simulink model "E010A5_C0_baseline_40A_1A_20260630"  (R2024b)
settings: Solver=VariableStepAuto  StartTime=0.0  StopTime=0.54e-3  MaxStep=5e-9  RelTol=1e-3
undefined symbols (not defined in the file): A_init, A_lower, A_upper, Cout, DCR_L1, DCR_L2, DCR_L3, DCR_L4, E010A5_DeltaI_Drop_Threshold_High, E010A5_IL_Sense_Gain1, E010A5_IL_Sense_Gain2, E010A5_IL_Sense_Gain3, E010A5_IL_Sense_Gain4, ESR_C, IdealIQCOT_Enable, IL_adc_counts_per_A, IL_pk_limit_adc_neg, IL_pk_limit_adc_pos, Iload_final, Iload_initial, Iph, Iqcot_enable, kappa_cmd, Kiqcot, Kvc_iqcot, L, Lambda0_iqcot, Lambda_m2, rho_cmd, Ri_iqcot, t_load_step, Tblank, Tdead, Tiqcot_leak, Toff_min, Ton_cmd, Ton_iq_max, Ton_iq_min, Ts_ctrl, Tslot, Tss, Vc_bias_iqcot, Vcot_ramp_amp, Vcot_ramp_enable, Vhys, Vin, Vo_ref
libraries: simulink x29, spsCurrentMeasurementLib x8, spsMosfetLib x8, spsSeriesRLCBranchLib x5, spsVoltageMeasurementLib x5, spsDCVoltageSourceLib x4, spsControlledCurrentSourceLib x1, spsGroundLib x1, spspowerguiLib x1
(part 1 of 2)
settings Model: Creator=zengruize  LastModifiedBy=zengruize

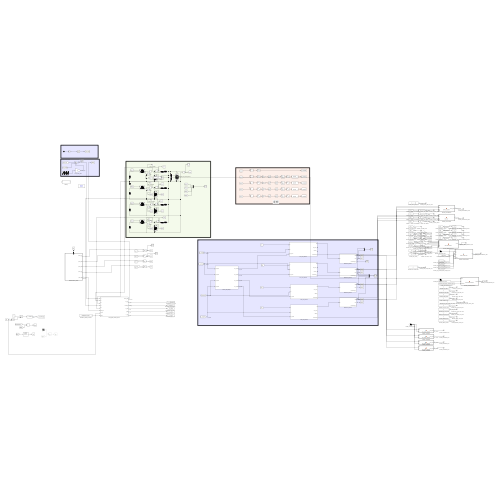
[thumbnail: Simulink's stored preview of the top-level diagram]
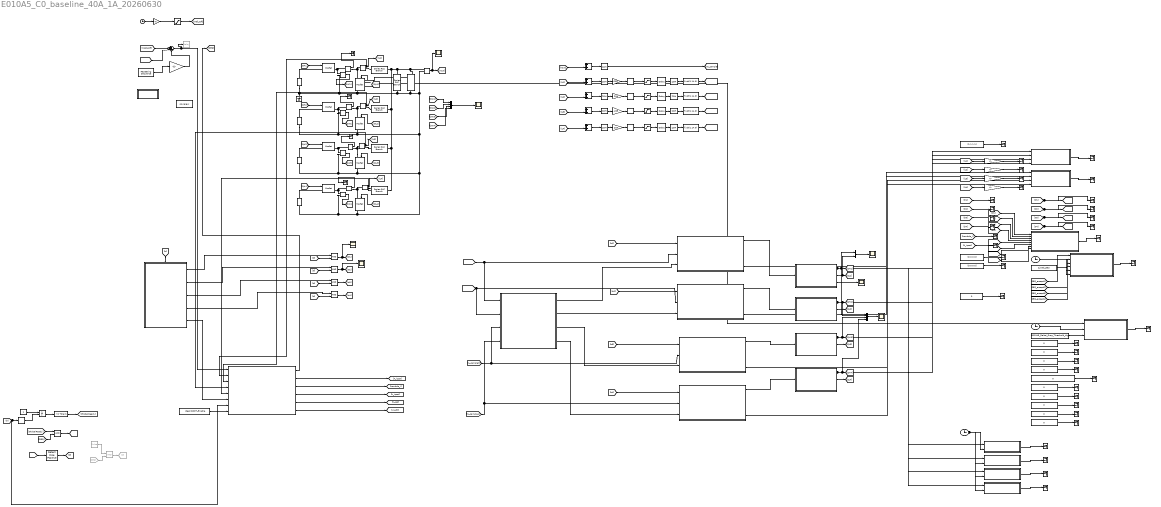
== system E010A5_C0_baseline_40A_1A_20260630 ==
  note: cot
  note: 输出电压误差比较器
  note: 功率级
  note: 软启动
  note: 采样
  Add{,1..4} (5 alike) : Sum
  Bus Creator : BusCreator  Inputs=4
  Bus Creator1 : BusCreator  Inputs=2
  Bus Creator2 : BusCreator  Inputs=4
  COT_Cell_1Phase1 : Subsystem
  COT_Cell_1Phase2 : Subsystem
  COT_Cell_1Phase3 : Subsystem
  COT_Cell_1Phase4 : Subsystem
  Clock : Clock
  Compare To Constant : simulink/Logic and Bit Operations/Compare To Constant  relop=>=  const=Tblank  OutDataTypeStr=boolean
  Constant : Constant
  Current Measurement{,1..3} (4 alike) : spsCurrentMeasurementLib/Current Measurement  PhasorSimulation=off  OutputType=Complex  PSBequivalent=0
  DC Voltage Source{,1..3} (4 alike) : spsDCVoltageSourceLib/DC Voltage Source  Amplitude=Vin  Measurements=None
  Data Type Conversion{,2..4} (4 alike) : DataTypeConversion  OutDataTypeStr=fixdt(1,14,0)  SaturateOnIntegerOverflow=off  RndMeth=Floor
  Detect Rise Positive : simulink/Logic and Bit Operations/Detect Rise Positive  vinit=0  OutDataTypeStr=boolean
  E010A5_ActiveHSPhase : MATLAB Function  TreatAsAtomicUnit=on
  E010A5_ActiveHSPhase_Term : Terminator
  E010A5_CurrentLimitHit : MATLAB Function  TreatAsAtomicUnit=on
  E010A5_CurrentLimitHit_Term : Terminator
  E010A5_IL_Sense_Gain_Block1 : Gain  Gain=E010A5_IL_Sense_Gain1
  E010A5_IL_Sense_Gain_Block2 : Gain  Gain=E010A5_IL_Sense_Gain2
  E010A5_IL_Sense_Gain_Block3 : Gain  Gain=E010A5_IL_Sense_Gain3
  E010A5_IL_Sense_Gain_Block4 : Gain  Gain=E010A5_IL_Sense_Gain4
  E010A5_IL_Sense_Term{1..4} (4 alike) : Terminator
  E010A5_LoadCurrentStep : Step  Time=t_load_step  Before=Iload_initial  After=Iload_final  SampleTime=0
  E010A5_Load_Current_Source : spsControlledCurrentSourceLib/Controlled Current Source  Initialize=on  Source_Type=DC  Amplitude=0  Phase=0  Frequency=0  Measurements=None
  E010A5_Log_Lambda_i_Term : Terminator
  E010A5_Log_REQ1_Term : Terminator
  E010A5_Log_REQ2_Term : Terminator
  E010A5_Log_REQ3_Term : Terminator
  E010A5_Log_REQ4_Term : Terminator
  E010A5_Log_area_int_i_Term : Terminator
  E010A5_PhaseOrderError : MATLAB Function  TreatAsAtomicUnit=on  SystemSampleTime=Ts_ctrl
  E010A5_PhaseOrderError_Term : Terminator
  E010A5_PhaseOrder_Clock : Clock
  E010A5_PhaseOrder_LoadStepTime : Constant  Value=t_load_step
  E010A5_REQAccept_Term{1..4} (4 alike) : Terminator
  E010A5_REQRejectReason : MATLAB Function  TreatAsAtomicUnit=on
  E010A5_REQRejectReason_Term : Terminator
  E010A5_SevereDropDetector : MATLAB Function  TreatAsAtomicUnit=on  SystemSampleTime=Ts_ctrl
  E010A5_SevereDropDetector_Clock : Clock
  E010A5_SevereDropDetector_Term : Terminator
  E010A5_SevereDropThreshold : Constant  Value=E010A5_DeltaI_Drop_Threshold_High
  E010A5_TonActual1 : MATLAB Function  TreatAsAtomicUnit=on  SystemSampleTime=Ts_ctrl
  E010A5_TonActual1_Term : Terminator
  E010A5_TonActual2 : MATLAB Function  TreatAsAtomicUnit=on  SystemSampleTime=Ts_ctrl
  E010A5_TonActual2_Term : Terminator
  E010A5_TonActual3 : MATLAB Function  TreatAsAtomicUnit=on  SystemSampleTime=Ts_ctrl
  E010A5_TonActual3_Term : Terminator
  E010A5_TonActual4 : MATLAB Function  TreatAsAtomicUnit=on  SystemSampleTime=Ts_ctrl
  E010A5_TonActual4_Term : Terminator
  E010A5_TonActual_Clock : Clock
  E010A5_Ton_saved_i : Constant  Value=[0 0 0 0]
  E010A5_Ton_saved_i_Term : Terminator
  E010A5_Ton_trunc_i : Constant  Value=[0 0 0 0]
  E010A5_Ton_trunc_i_Term : Terminator
  E010A5_a_O_state : Constant  Value=0
  E010A5_a_O_state_Term : Terminator
  E010A5_active_phase_set : Constant  Value=[1 1 1 1]
  E010A5_active_phase_set_Term : Terminator
  E010A5_area_bleed_count : Constant  Value=0
  E010A5_area_bleed_count_Term : Terminator
  E010A5_area_hold_count : Constant  Value=0
  E010A5_area_hold_count_Term : Terminator
  E010A5_area_hold_state : Constant  Value=0
  E010A5_area_hold_state_Term : Terminator
  E010A5_area_reset_count : Constant  Value=0
  E010A5_area_reset_count_Term : Terminator
  E010A5_burst_pulse_count_after_reentry : Constant  Value=0
  E010A5_burst_pulse_count_after_reentry_Term : Terminator
  E010A5_fallback_count : Constant  Value=0
  E010A5_fallback_count_Term : Terminator
  E010A5_fallback_reason : Constant  Value=0
  E010A5_fallback_reason_Term : Terminator
  E010A5_fallback_state : Constant  Value=0
  E010A5_fallback_state_Term : Terminator
  E010A5_pulse_inhibit_state : Constant  Value=0
  E010A5_pulse_inhibit_state_Term : Terminator
  E010A5_reentry_state : Constant  Value=0
  E010A5_reentry_state_Term : Terminator
  From31 : From  Commented=on  GotoTag=REQ
  Gain : Gain  Gain=Vo_ref / Tss
  Gain11 : Gain  Gain=205
  Gain12 : Gain  Gain=-205
  Gain13 : Gain  Gain=205
  Gain9 : Gain  Gain=-205
  GateDriver_1Phase1 : Subsystem
  GateDriver_1Phase2 : Subsystem
  GateDriver_1Phase3 : Subsystem
  GateDriver_1Phase4 : Subsystem
  Goto26 : Goto  Commented=on  GotoTag=tr
  Ground : spsGroundLib/Ground  LConnTagsString=a
  IHS_Terminator{1..4} (4 alike) : Terminator
  IL_Measurement{1..4} (4 alike) : spsCurrentMeasurementLib/Current Measurement  PhasorSimulation=off  OutputType=Complex  PSBequivalent=0
  IQCOT_Ton_Adapter : Subsystem
  IdealIQCOT_Enable_Constant : Constant  Value=IdealIQCOT_Enable
  Ideal_Digital_IQCOT_Request : Subsystem
  Integrator : Integrator  ExternalReset=rising
  Logical Operator{,1..4} (5 alike) : Logic  AllPortsSameDT=off  OutDataTypeStr=boolean
  Logical Operator5 : Logic  Commented=on  AllPortsSameDT=off  OutDataTypeStr=boolean
  Memory : Memory
  Mosfet{,1..3} (4 alike) : spsMosfetLib/Mosfet  Ron=Ron_HS  Lon=0  Rd=Rd_body  Vfd=Vfd_body  IC=0  Rs=Rs_snubber  Cs=Cs_snubber  Measurements=on
  Mosfet{4..7} (4 alike) : spsMosfetLib/Mosfet  Ron=Ron_LS  Lon=0  Rd=Rd_body  Vfd=Vfd_body  IC=0  Rs=Rs_snubber  Cs=Cs_snubber  Measurements=on
  OnDelay : Subsystem
  PhaseScheduler_4Phase : Subsystem  TreatAsAtomicUnit=on
  Pulse Generator : DiscretePulseGenerator  Commented=on  PulseType=Time based  Period=Tblank  PulseWidth=5
  Quantizer{1..4} (4 alike) : Quantizer  QuantizationInterval=1
  Relay : Relay  Commented=through  OnSwitchValue=Vhys/2  OffSwitchValue=-Vhys/2
  Saturation{,1,3..4} (4 alike) : Saturate  UpperLimit=8191  LowerLimit=-8191
  Saturation2 : Saturate  UpperLimit=Vo_ref  LowerLimit=0
  Scope{,1..6} (7 alike) : Scope
  Series RLC Branch : spsSeriesRLCBranchLib/Series RLC Branch  LConnTagsString=__new0  RConnTagsString=__new0  BranchType=RL  Resistance=DCR_L1  Inductance=L  SetiL0=off  InitialCurrent=0  Capacitance=1e-6  Setx0=off  InitialVoltage=0  Measurements=None
  Series RLC Branch1 : spsSeriesRLCBranchLib/Series RLC Branch  LConnTagsString=__new0  RConnTagsString=__new0  BranchType=RL  Resistance=DCR_L2  Inductance=L  SetiL0=off  InitialCurrent=0  Capacitance=1e-6  Setx0=off  InitialVoltage=0  Measurements=None
  Series RLC Branch2 : spsSeriesRLCBranchLib/Series RLC Branch  LConnTagsString=__new0  RConnTagsString=__new0  BranchType=RL  Resistance=DCR_L3  Inductance=L  SetiL0=off  InitialCurrent=0  Capacitance=1e-6  Setx0=off  InitialVoltage=0  Measurements=None
  Series RLC Branch3 : spsSeriesRLCBranchLib/Series RLC Branch  LConnTagsString=__new0  RConnTagsString=__new0  BranchType=RL  Resistance=DCR_L4  Inductance=L  SetiL0=off  InitialCurrent=0  Capacitance=1e-6  Setx0=off  InitialVoltage=0  Measurements=None
  Series RLC Branch4 : spsSeriesRLCBranchLib/Series RLC Branch  LConnTagsString=__new0  RConnTagsString=__new0  BranchType=RC  Resistance=ESR_C  Inductance=1e-3  SetiL0=off  InitialCurrent=0  Capacitance=Cout  Setx0=on  InitialVoltage=Vo_ref  Measurements=None
  Sum : Sum  Inputs=|+--
  Transport Delay{1..4} (4 alike) : TransportDelay  DelayTime=5/25000000
  VCOT_Ramp_Gain : Gain  Gain=Vcot_ramp_enable * Vcot_ramp_amp
  VCOT_Ramp_Unit : simulink/Sources/Repeating Sequence  rep_seq_t=[0 Tslot]  rep_seq_y=[0 1]
  Voltage Measurement{,1..4} (5 alike) : spsVoltageMeasurementLib/Voltage Measurement  PhasorSimulation=off  OutputType=Complex  PSBequivalent=0
  Zero-Order Hold{1..4,19..23} (9 alike) : ZeroOrderHold  SampleTime=1/25000000
  powergui : spspowerguiLib/powergui  Priority=1  SimulationMode=Discrete  SampleTime=2e-9  frequency=60  Iterations=50  frequencyindice=0  Pbase=100e6  ErrMax=1e-4  UnitsV=kV  UnitsW=MW  buscounter=0  FunctionMessages=off  echomessages=off  EnableUseOfTLC=off  CurrentSourceSwitches=off  DisableSnubberDevices=off  DisableRonSwitches=off  DisableVfSwitches=off  DisplayEquations=off  AutomaticDiscreteSolvers=off  SolverType=Tustin/Backward Euler (TBE)  Interpol=off  ExternalGateDelay=off  methode=off  Ts=100  x0status=blocks  SPID=on  SwTol=0  HookPort=off  NonlinearTolerance=1e-4  nMaxIteration=100  ContinueOnMaxIteration=off  RestoreLinks=warning  ResistiveCurrentMeasurement=off  Frange=[0:2:500]  Ylog=off  Xlog=on  ShowGrid=off  save=off  variable=ZData  structure=0  ZoomFFT=off  StartTime=0.0  cycles=1  DisplayStyle=1  fundamental=60  FreqAxis=off  MaxFrequency=1000  frequencyindicesteady=1  RmsSteady=1  display=off
  wires:
  [QH1] -> Mosfet/1
  [QH4] -> Mosfet3/1
  [QH2] -> Mosfet1/1
  [QH3] -> Mosfet2/1
  [QL1] -> Mosfet4/1
  [QL2] -> Mosfet5/1
  [QL3] -> Mosfet6/1
  [QL4] -> Mosfet7/1
  Voltage Measurement2/1 -> [SW2]  "SW2"
  Voltage Measurement3/1 -> [SW3]  "SW3"
  Voltage Measurement1/1 -> [SW1]  "SW1"
  Voltage Measurement4/1 -> [SW4]  "SW4"
  GateDriver_1Phase1/1(QHi) -> Bus Creator1/1, [QH1], Bus Creator2/1, E010A5_ActiveHSPhase/1(qh1), E010A5_TonActual1/1(qh)  "QH1"
  GateDriver_1Phase2/1(QHi) -> Bus Creator2/2, [QH2], E010A5_ActiveHSPhase/2(qh2), E010A5_TonActual2/1(qh)  "QH2"
  GateDriver_1Phase3/1(QHi) -> Bus Creator2/3, [QH3], E010A5_ActiveHSPhase/3(qh3), E010A5_TonActual3/1(qh)  "QH3"
  GateDriver_1Phase4/1(QHi) -> Bus Creator2/4, [QH4], E010A5_ActiveHSPhase/4(qh4), E010A5_TonActual4/1(qh)  "QH4"
  GateDriver_1Phase1/2(QLi) -> Bus Creator1/2, [QL1]  "QL1"
  GateDriver_1Phase2/2(QLi) -> [QL2]  "QL2"
  GateDriver_1Phase3/2(QLi) -> [QL3]  "QL3"
  GateDriver_1Phase4/2(QLi) -> [QL4]  "QL4"
  COT_Cell_1Phase1/1(Qi) -> GateDriver_1Phase1/1(Qi)
  COT_Cell_1Phase2/1(Qi) -> GateDriver_1Phase2/1(Qi)
  COT_Cell_1Phase3/1(Qi) -> GateDriver_1Phase3/1(Qi)
  COT_Cell_1Phase4/1(Qi) -> GateDriver_1Phase4/1(Qi)
  GateDriver_1Phase1/3(ShootThrough_i) -> Scope1/1
  Bus Creator/1 -> Scope2/1
  [SW1] -> Bus Creator/1
  [SW2] -> Bus Creator/2
  [SW3] -> Bus Creator/3
  [SW4] -> Bus Creator/4
  Bus Creator1/1 -> Scope3/1
  Saturation2/1 -> [Vref_soft]
  Gain/1 -> Saturation2/1
  Clock/1 -> Gain/1
  Voltage Measurement/1 -> Scope/1, [Vout]  "Vout"
  [Vref_soft] -> Sum/1
  [Vo_sample] -> Sum/2
  Sum/1 -> Ideal_Digital_IQCOT_Request/1(e_v), Relay/1  "e_v"
  Constant/1 -> Integrator/1
  Integrator/1 -> Compare To Constant/1
  Compare To Constant/1 -> [GlobalReady]  "Allow"
  [GlobalReady] -> Logical Operator/1
  [REQ] -> Logical Operator/2
  Logical Operator/1 -> [Allow]
  [Allow] -> Detect Rise Positive/1
  Detect Rise Positive/1 -> [tr]
  [tr] -> PhaseScheduler_4Phase/Trigger  "tr"
  PhaseScheduler_4Phase/1(phase_en1) -> Logical Operator1/1
  [tr] -> Logical Operator1/2
  PhaseScheduler_4Phase/2(phase_en2) -> Logical Operator2/1
  [tr] -> Logical Operator2/2
  PhaseScheduler_4Phase/3(phase_en3) -> Logical Operator3/1
  [tr] -> Logical Operator3/2
  PhaseScheduler_4Phase/4(phase_en4) -> Logical Operator4/1
  [tr] -> Logical Operator4/2
  Logical Operator1/1 -> Scope4/1, [tr1]  "tr1"
  Logical Operator2/1 -> Scope5/1, [tr2]  "tr2"
  Logical Operator3/1 -> [tr3]  "tr3"
  Logical Operator4/1 -> [tr4]  "tr4"
  [tr1] -> COT_Cell_1Phase1/1(tri)
  [tr2] -> COT_Cell_1Phase2/1(tri)
  [tr3] -> COT_Cell_1Phase3/1(tri)
  [tr4] -> COT_Cell_1Phase4/1(tri)
  [IL_sample1] -> COT_Cell_1Phase1/2(ILi), IQCOT_Ton_Adapter/1(IL_sample1)  "IL_sample1"
  [IL_sample2] -> IQCOT_Ton_Adapter/2(IL_sample2), COT_Cell_1Phase2/2(ILi)  "IL_sample2"
  [IL_sample3] -> IQCOT_Ton_Adapter/3(IL_sample3), COT_Cell_1Phase3/2(ILi)  "IL_sample3"
  [IL_sample4] -> IQCOT_Ton_Adapter/4(IL_sample4), COT_Cell_1Phase4/2(ILi)  "IL_sample4"
  [tr] -> Memory/1, Ideal_Digital_IQCOT_Request/7(tr_reset)  "tr_reset"
  Memory/1 -> Integrator/2
  Logical Operator5/1 -> Goto26/1
  Pulse Generator/1 -> Logical Operator5/1
  From31/1 -> Logical Operator5/2
  Bus Creator2/1 -> Scope6/1
  IL_Measurement1/1 -> [IL1], Ideal_Digital_IQCOT_Request/2(IL1)  "IL1"
  IL_Measurement2/1 -> [IL2], Ideal_Digital_IQCOT_Request/3(IL2)  "IL2"
  IL_Measurement3/1 -> [IL3], Ideal_Digital_IQCOT_Request/4(IL3)  "IL3"
  IL_Measurement4/1 -> [IL4], Ideal_Digital_IQCOT_Request/5(IL4)  "IL4"
  Current Measurement/1 -> IHS_Terminator1/1
  Current Measurement1/1 -> IHS_Terminator2/1
  Current Measurement2/1 -> IHS_Terminator3/1
  Current Measurement3/1 -> IHS_Terminator4/1
  Zero-Order Hold23/1 -> Gain13/1
  Zero-Order Hold20/1 -> Gain9/1
  Zero-Order Hold3/1 -> Data Type Conversion3/1
  Zero-Order Hold4/1 -> Data Type Conversion2/1
  Saturation4/1 -> Transport Delay4/1
  Zero-Order Hold1/1 -> Data Type Conversion/1
  [IL3] -> Add3/2
  Add3/1 -> Zero-Order Hold22/1
  Quantizer1/1 -> Saturation/1
  Quantizer4/1 -> Saturation4/1
  Gain12/1 -> Quantizer3/1
  [IL4] -> Add4/2
  Add/1 -> Zero-Order Hold19/1
  Data Type Conversion/1 -> [IL_sample1]
  Data Type Conversion2/1 -> [IL_sample4]
  Add4/1 -> Zero-Order Hold23/1
  Transport Delay3/1 -> Zero-Order Hold3/1
  Saturation3/1 -> Transport Delay3/1
  Add1/1 -> Zero-Order Hold20/1
  [IL1] -> Add1/2
  Transport Delay4/1 -> Zero-Order Hold4/1
  Zero-Order Hold21/1 -> Gain11/1
  Data Type Conversion3/1 -> [IL_sample3]
  Gain9/1 -> Quantizer1/1
  Gain11/1 -> Quantizer2/1
  Saturation/1 -> Transport Delay1/1
  [IL2] -> Add2/2
  Transport Delay2/1 -> Zero-Order Hold2/1
  Zero-Order Hold19/1 -> [Vo_sample]
  Gain13/1 -> Quantizer4/1
  Quantizer3/1 -> Saturation3/1
  Data Type Conversion4/1 -> [IL_sample2]
  Zero-Order Hold2/1 -> Data Type Conversion4/1
  Add2/1 -> Zero-Order Hold21/1
  Transport Delay1/1 -> Zero-Order Hold1/1
  [Vout] -> Add/2
  Saturation1/1 -> Transport Delay2/1
  Zero-Order Hold22/1 -> Gain12/1
  Quantizer2/1 -> Saturation1/1
  VCOT_Ramp_Unit/1 -> VCOT_Ramp_Gain/1
  VCOT_Ramp_Gain/1 -> Sum/3  "Vcot_ramp"
  IQCOT_Ton_Adapter/1(Ton_iqcot1) -> COT_Cell_1Phase1/3(Ton_iqcot1)  "Ton_cmd1"
  IQCOT_Ton_Adapter/2(Ton_iqcot2) -> COT_Cell_1Phase2/3(Ton_iqcot2)  "Ton_cmd2"
  IQCOT_Ton_Adapter/3(Ton_iqcot3) -> COT_Cell_1Phase3/3(Ton_iqcot3)  "Ton_cmd3"
  IQCOT_Ton_Adapter/4(Ton_iqcot4) -> COT_Cell_1Phase4/3(Ton_iqcot4)  "Ton_cmd4"
  PhaseScheduler_4Phase/5(phase_idx) -> Ideal_Digital_IQCOT_Request/6(phase_idx)  "phase_idx"
  IdealIQCOT_Enable_Constant/1 -> Ideal_Digital_IQCOT_Request/8(enable)
  Ideal_Digital_IQCOT_Request/1(REQ_iqcot) -> [REQ]  "REQ_iqcot"
  Ideal_Digital_IQCOT_Request/2(A_iqcot) -> [A_iqcot]  "A_iqcot"
  Ideal_Digital_IQCOT_Request/3(Lambda_i) -> [Lambda_i]  "Lambda_i"
  Ideal_Digital_IQCOT_Request/4(h_iqcot) -> [h_iqcot]  "h_iqcot"
  Ideal_Digital_IQCOT_Request/5(IL_sel) -> [IL_sel]  "IL_sel"
  Ideal_Digital_IQCOT_Request/6(vc_ctrl) -> [vc_ctrl]  "vc_ctrl"
  E010A5_LoadCurrentStep/1 -> E010A5_Load_Current_Source/1, E010A5_SevereDropDetector/1(iload)  "Iload"
  E010A5_active_phase_set/1 -> E010A5_active_phase_set_Term/1  "active_phase_set"
  [IL1] -> E010A5_IL_Sense_Gain_Block1/1
  E010A5_IL_Sense_Gain_Block1/1 -> E010A5_IL_Sense_Term1/1  "IL_sense1"
  [IL2] -> E010A5_IL_Sense_Gain_Block2/1
  E010A5_IL_Sense_Gain_Block2/1 -> E010A5_IL_Sense_Term2/1  "IL_sense2"
  [IL3] -> E010A5_IL_Sense_Gain_Block3/1
  E010A5_IL_Sense_Gain_Block3/1 -> E010A5_IL_Sense_Term3/1  "IL_sense3"
  [IL4] -> E010A5_IL_Sense_Gain_Block4/1
  E010A5_IL_Sense_Gain_Block4/1 -> E010A5_IL_Sense_Term4/1  "IL_sense4"
  [tr1] -> E010A5_Log_REQ1_Term/1  "REQ1"
  [tr2] -> E010A5_Log_REQ2_Term/1  "REQ2"
  [tr3] -> E010A5_Log_REQ3_Term/1  "REQ3"
  [tr4] -> E010A5_Log_REQ4_Term/1  "REQ4"
  [Lambda_i] -> E010A5_Log_Lambda_i_Term/1  "Lambda_i"
  [A_iqcot] -> E010A5_Log_area_int_i_Term/1  "area_int_i"
  E010A5_ActiveHSPhase/1(active_phase) -> E010A5_ActiveHSPhase_Term/1  "active_HS_phase"
  COT_Cell_1Phase1/4(CurrentLimit_i) -> E010A5_CurrentLimitHit/1(u1)
  COT_Cell_1Phase2/4(CurrentLimit_i) -> E010A5_CurrentLimitHit/2(u2)
  COT_Cell_1Phase3/4(CurrentLimit_i) -> E010A5_CurrentLimitHit/3(u3)
  COT_Cell_1Phase4/4(CurrentLimit_i) -> E010A5_CurrentLimitHit/4(u4)
  E010A5_CurrentLimitHit/1(y) -> E010A5_CurrentLimitHit_Term/1  "current_limit_hit"
  [tr1] -> [REQ_accept1], E010A5_REQAccept_Term1/1  "REQ_accept1"
  [tr2] -> [REQ_accept2], E010A5_REQAccept_Term2/1  "REQ_accept2"
  [tr3] -> [REQ_accept3], E010A5_REQAccept_Term3/1  "REQ_accept3"
  [tr4] -> [REQ_accept4], E010A5_REQAccept_Term4/1  "REQ_accept4"
  E010A5_Ton_trunc_i/1 -> E010A5_Ton_trunc_i_Term/1  "Ton_trunc_i"
  E010A5_Ton_saved_i/1 -> E010A5_Ton_saved_i_Term/1  "Ton_saved_i"
  E010A5_pulse_inhibit_state/1 -> E010A5_pulse_inhibit_state_Term/1  "pulse_inhibit_state"
  [tr1] -> E010A5_REQRejectReason/1(r1)
  [REQ_accept1] -> E010A5_REQRejectReason/5(a1)
  [tr2] -> E010A5_REQRejectReason/2(r2)
  [REQ_accept2] -> E010A5_REQRejectReason/6(a2)
  [tr3] -> E010A5_REQRejectReason/3(r3)
  [REQ_accept3] -> E010A5_REQRejectReason/7(a3)
  [tr4] -> E010A5_REQRejectReason/4(r4)
  [REQ_accept4] -> E010A5_REQRejectReason/8(a4)
  E010A5_REQRejectReason/1(reason) -> E010A5_REQRejectReason_Term/1  "REQ_reject_reason"
  [REQ_accept1] -> E010A5_PhaseOrderError/1(a1)
  [REQ_accept2] -> E010A5_PhaseOrderError/2(a2)
  [REQ_accept3] -> E010A5_PhaseOrderError/3(a3)
  [REQ_accept4] -> E010A5_PhaseOrderError/4(a4)
  E010A5_PhaseOrder_Clock/1 -> E010A5_PhaseOrderError/5(t)
  E010A5_PhaseOrder_LoadStepTime/1 -> E010A5_PhaseOrderError/6(t_step)
  E010A5_PhaseOrderError/1(err) -> E010A5_PhaseOrderError_Term/1  "phase_order_error"
  E010A5_SevereDropDetector_Clock/1 -> E010A5_SevereDropDetector/2(t)
  E010A5_SevereDropThreshold/1 -> E010A5_SevereDropDetector/3(threshold)
  E010A5_SevereDropDetector/1(detected) -> E010A5_SevereDropDetector_Term/1  "severe_drop_detected"
  E010A5_a_O_state/1 -> E010A5_a_O_state_Term/1  "a_O_state"
  E010A5_area_hold_state/1 -> E010A5_area_hold_state_Term/1  "area_hold_state"
  E010A5_reentry_state/1 -> E010A5_reentry_state_Term/1  "reentry_state"
  E010A5_fallback_state/1 -> E010A5_fallback_state_Term/1  "fallback_state"
  E010A5_burst_pulse_count_after_reentry/1 -> E010A5_burst_pulse_count_after_reentry_Term/1  "burst_pulse_count_after_reentry"
  E010A5_area_hold_count/1 -> E010A5_area_hold_count_Term/1  "area_hold_count"
  E010A5_area_reset_count/1 -> E010A5_area_reset_count_Term/1  "area_reset_count"
  E010A5_area_bleed_count/1 -> E010A5_area_bleed_count_Term/1  "area_bleed_count"
  E010A5_fallback_count/1 -> E010A5_fallback_count_Term/1  "fallback_count"
  E010A5_fallback_reason/1 -> E010A5_fallback_reason_Term/1  "fallback_reason"
  E010A5_TonActual_Clock/1 -> E010A5_TonActual1/2(t), E010A5_TonActual2/2(t), E010A5_TonActual3/2(t), E010A5_TonActual4/2(t)
  E010A5_TonActual1/1(Ton_actual) -> E010A5_TonActual1_Term/1  "Ton_actual1"
  E010A5_TonActual2/1(Ton_actual) -> E010A5_TonActual2_Term/1  "Ton_actual2"
  E010A5_TonActual3/1(Ton_actual) -> E010A5_TonActual3_Term/1  "Ton_actual3"
  E010A5_TonActual4/1(Ton_actual) -> E010A5_TonActual4_Term/1  "Ton_actual4"
  connections:
  DC Voltage Source/LConn1 -- Voltage Measurement1/LConn2 -- Mosfet7/RConn1 -- Voltage Measurement4/LConn2 -- DC Voltage Source3/LConn1 -- Mosfet6/RConn1 -- Voltage Measurement3/LConn2 -- DC Voltage Source2/LConn1 -- DC Voltage Source1/LConn1 -- Voltage Measurement2/LConn2 -- Mosfet5/RConn1 -- Voltage Measurement/LConn2 -- E010A5_Load_Current_Source/RConn1 -- Series RLC Branch4/RConn1 -- Mosfet4/RConn1 -- Ground/LConn1
  Mosfet/LConn1 -- DC Voltage Source/RConn1
  DC Voltage Source1/RConn1 -- Mosfet1/LConn1
  Mosfet1/RConn1 -- Current Measurement1/LConn1 -- Voltage Measurement2/LConn1
  DC Voltage Source2/RConn1 -- Mosfet2/LConn1
  Mosfet2/RConn1 -- Current Measurement2/LConn1 -- Voltage Measurement3/LConn1
  DC Voltage Source3/RConn1 -- Mosfet3/LConn1
  Series RLC Branch/RConn1 -- Series RLC Branch3/RConn1 -- Series RLC Branch2/RConn1 -- Series RLC Branch1/RConn1 -- Voltage Measurement/LConn1 -- E010A5_Load_Current_Source/LConn1 -- Series RLC Branch4/LConn1
  Mosfet/RConn1 -- Current Measurement/LConn1 -- Voltage Measurement1/LConn1
  Mosfet3/RConn1 -- Current Measurement3/LConn1 -- Voltage Measurement4/LConn1
  Current Measurement/RConn1 -- Mosfet4/LConn1 -- IL_Measurement1/LConn1
  IL_Measurement1/RConn1 -- Series RLC Branch/LConn1
  Current Measurement1/RConn1 -- Mosfet5/LConn1 -- IL_Measurement2/LConn1
  IL_Measurement2/RConn1 -- Series RLC Branch1/LConn1
  Mosfet6/LConn1 -- Current Measurement2/RConn1 -- IL_Measurement3/LConn1
  IL_Measurement3/RConn1 -- Series RLC Branch2/LConn1
  Current Measurement3/RConn1 -- Mosfet7/LConn1 -- IL_Measurement4/LConn1
  IL_Measurement4/RConn1 -- Series RLC Branch3/LConn1

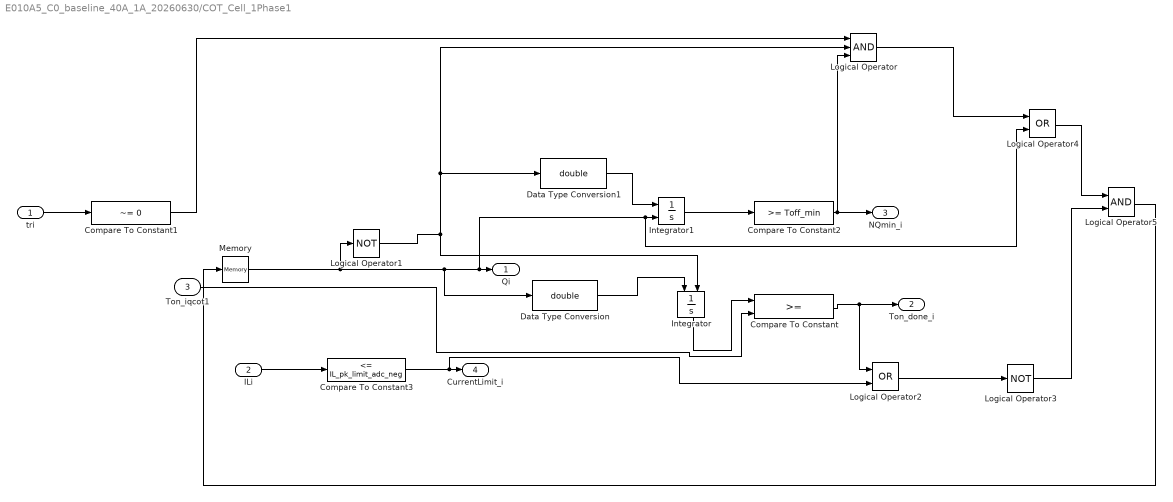
== system E010A5_C0_baseline_40A_1A_20260630/COT_Cell_1Phase1 ==
  tri : Inport
  ILi : Inport  Port=2
  Ton_iqcot1 : Inport  Port=3
  Compare To Constant : RelationalOperator  OutDataTypeStr=boolean  RndMeth=Simplest  InputSameDT=off
  Compare To Constant1 : simulink/Logic and Bit Operations/Compare To Constant  relop=~=  const=0  OutDataTypeStr=boolean
  Compare To Constant2 : simulink/Logic and Bit Operations/Compare To Constant  relop=>=  const=Toff_min  OutDataTypeStr=boolean
  Compare To Constant3 : simulink/Logic and Bit Operations/Compare To Constant  relop=<=  const=IL_pk_limit_adc_neg  OutDataTypeStr=boolean
  Data Type Conversion : DataTypeConversion  OutDataTypeStr=double  SaturateOnIntegerOverflow=off  RndMeth=Floor
  Data Type Conversion1 : DataTypeConversion  OutDataTypeStr=double  SaturateOnIntegerOverflow=off  RndMeth=Floor
  Integrator : Integrator  ExternalReset=level
  Integrator1 : Integrator  ExternalReset=level  InitialCondition=Toff_min
  Logical Operator : Logic  Inputs=3  AllPortsSameDT=off  OutDataTypeStr=boolean
  Logical Operator1 : Logic  Operator=NOT  AllPortsSameDT=off  OutDataTypeStr=boolean
  Logical Operator2 : Logic  Operator=OR  AllPortsSameDT=off  OutDataTypeStr=boolean
  Logical Operator3 : Logic  Operator=NOT  Inputs=3  AllPortsSameDT=off  OutDataTypeStr=boolean
  Logical Operator4 : Logic  Operator=OR  AllPortsSameDT=off  OutDataTypeStr=boolean
  Logical Operator5 : Logic  AllPortsSameDT=off  OutDataTypeStr=boolean
  Memory : Memory
  Qi : Outport
  Ton_done_i : Outport  Port=2
  NQmin_i : Outport  Port=3
  CurrentLimit_i : Outport  Port=4
  wires:
  Compare To Constant/1 -> Logical Operator2/1, Ton_done_i/1
  tri/1 -> Compare To Constant1/1
  Compare To Constant1/1 -> Logical Operator/1
  Memory/1 -> Logical Operator1/1, Data Type Conversion/1, Logical Operator4/2, Integrator1/2, Qi/1
  Logical Operator1/1 -> Data Type Conversion1/1, Logical Operator/2, Integrator/2
  Data Type Conversion/1 -> Integrator/1
  Integrator/1 -> Compare To Constant/1
  Data Type Conversion1/1 -> Integrator1/1
  Integrator1/1 -> Compare To Constant2/1
  Compare To Constant2/1 -> Logical Operator/3, NQmin_i/1
  ILi/1 -> Compare To Constant3/1
  Compare To Constant3/1 -> Logical Operator2/2, CurrentLimit_i/1
  Logical Operator2/1 -> Logical Operator3/1
  Logical Operator/1 -> Logical Operator4/1
  Logical Operator4/1 -> Logical Operator5/1
  Logical Operator3/1 -> Logical Operator5/2
  Logical Operator5/1 -> Memory/1
  Ton_iqcot1/1 -> Compare To Constant/2

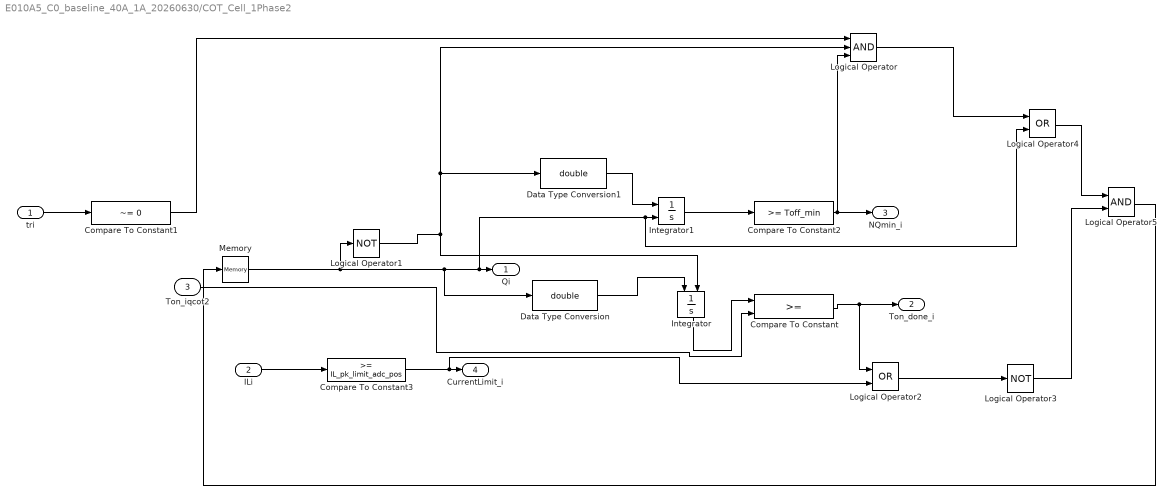
== system E010A5_C0_baseline_40A_1A_20260630/COT_Cell_1Phase2 ==
  tri : Inport
  ILi : Inport  Port=2
  Ton_iqcot2 : Inport  Port=3
  Compare To Constant : RelationalOperator  OutDataTypeStr=boolean  RndMeth=Simplest  InputSameDT=off
  Compare To Constant1 : simulink/Logic and Bit Operations/Compare To Constant  relop=~=  const=0  OutDataTypeStr=boolean
  Compare To Constant2 : simulink/Logic and Bit Operations/Compare To Constant  relop=>=  const=Toff_min  OutDataTypeStr=boolean
  Compare To Constant3 : simulink/Logic and Bit Operations/Compare To Constant  relop=>=  const=IL_pk_limit_adc_pos  OutDataTypeStr=boolean
  Data Type Conversion : DataTypeConversion  OutDataTypeStr=double  SaturateOnIntegerOverflow=off  RndMeth=Floor
  Data Type Conversion1 : DataTypeConversion  OutDataTypeStr=double  SaturateOnIntegerOverflow=off  RndMeth=Floor
  Integrator : Integrator  ExternalReset=level
  Integrator1 : Integrator  ExternalReset=level  InitialCondition=Toff_min
  Logical Operator : Logic  Inputs=3  AllPortsSameDT=off  OutDataTypeStr=boolean
  Logical Operator1 : Logic  Operator=NOT  AllPortsSameDT=off  OutDataTypeStr=boolean
  Logical Operator2 : Logic  Operator=OR  AllPortsSameDT=off  OutDataTypeStr=boolean
  Logical Operator3 : Logic  Operator=NOT  Inputs=3  AllPortsSameDT=off  OutDataTypeStr=boolean
  Logical Operator4 : Logic  Operator=OR  AllPortsSameDT=off  OutDataTypeStr=boolean
  Logical Operator5 : Logic  AllPortsSameDT=off  OutDataTypeStr=boolean
  Memory : Memory
  Qi : Outport
  Ton_done_i : Outport  Port=2
  NQmin_i : Outport  Port=3
  CurrentLimit_i : Outport  Port=4
  wires:
  Compare To Constant/1 -> Logical Operator2/1, Ton_done_i/1
  tri/1 -> Compare To Constant1/1
  Compare To Constant1/1 -> Logical Operator/1
  Memory/1 -> Logical Operator1/1, Data Type Conversion/1, Logical Operator4/2, Integrator1/2, Qi/1
  Logical Operator1/1 -> Data Type Conversion1/1, Logical Operator/2, Integrator/2
  Data Type Conversion/1 -> Integrator/1
  Integrator/1 -> Compare To Constant/1
  Data Type Conversion1/1 -> Integrator1/1
  Integrator1/1 -> Compare To Constant2/1
  Compare To Constant2/1 -> Logical Operator/3, NQmin_i/1
  ILi/1 -> Compare To Constant3/1
  Compare To Constant3/1 -> Logical Operator2/2, CurrentLimit_i/1
  Logical Operator2/1 -> Logical Operator3/1
  Logical Operator/1 -> Logical Operator4/1
  Logical Operator4/1 -> Logical Operator5/1
  Logical Operator3/1 -> Logical Operator5/2
  Logical Operator5/1 -> Memory/1
  Ton_iqcot2/1 -> Compare To Constant/2

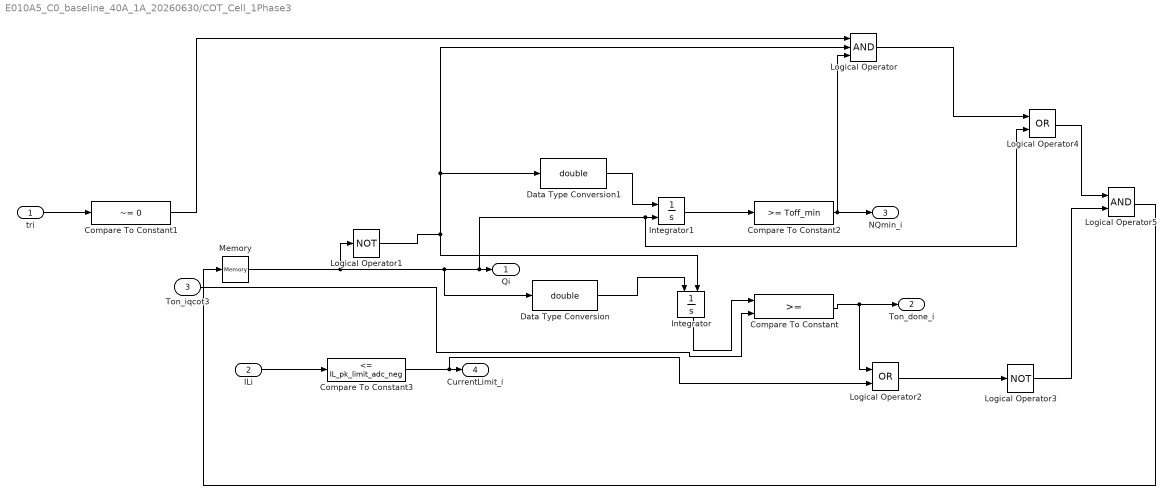
== system E010A5_C0_baseline_40A_1A_20260630/COT_Cell_1Phase3 ==
  tri : Inport
  ILi : Inport  Port=2
  Ton_iqcot3 : Inport  Port=3
  Compare To Constant : RelationalOperator  OutDataTypeStr=boolean  RndMeth=Simplest  InputSameDT=off
  Compare To Constant1 : simulink/Logic and Bit Operations/Compare To Constant  relop=~=  const=0  OutDataTypeStr=boolean
  Compare To Constant2 : simulink/Logic and Bit Operations/Compare To Constant  relop=>=  const=Toff_min  OutDataTypeStr=boolean
  Compare To Constant3 : simulink/Logic and Bit Operations/Compare To Constant  relop=<=  const=IL_pk_limit_adc_neg  OutDataTypeStr=boolean
  Data Type Conversion : DataTypeConversion  OutDataTypeStr=double  SaturateOnIntegerOverflow=off  RndMeth=Floor
  Data Type Conversion1 : DataTypeConversion  OutDataTypeStr=double  SaturateOnIntegerOverflow=off  RndMeth=Floor
  Integrator : Integrator  ExternalReset=level
  Integrator1 : Integrator  ExternalReset=level  InitialCondition=Toff_min
  Logical Operator : Logic  Inputs=3  AllPortsSameDT=off  OutDataTypeStr=boolean
  Logical Operator1 : Logic  Operator=NOT  AllPortsSameDT=off  OutDataTypeStr=boolean
  Logical Operator2 : Logic  Operator=OR  AllPortsSameDT=off  OutDataTypeStr=boolean
  Logical Operator3 : Logic  Operator=NOT  Inputs=3  AllPortsSameDT=off  OutDataTypeStr=boolean
  Logical Operator4 : Logic  Operator=OR  AllPortsSameDT=off  OutDataTypeStr=boolean
  Logical Operator5 : Logic  AllPortsSameDT=off  OutDataTypeStr=boolean
  Memory : Memory
  Qi : Outport
  Ton_done_i : Outport  Port=2
  NQmin_i : Outport  Port=3
  CurrentLimit_i : Outport  Port=4
  wires:
  Compare To Constant/1 -> Logical Operator2/1, Ton_done_i/1
  tri/1 -> Compare To Constant1/1
  Compare To Constant1/1 -> Logical Operator/1
  Memory/1 -> Logical Operator1/1, Data Type Conversion/1, Logical Operator4/2, Integrator1/2, Qi/1
  Logical Operator1/1 -> Data Type Conversion1/1, Logical Operator/2, Integrator/2
  Data Type Conversion/1 -> Integrator/1
  Integrator/1 -> Compare To Constant/1
  Data Type Conversion1/1 -> Integrator1/1
  Integrator1/1 -> Compare To Constant2/1
  Compare To Constant2/1 -> Logical Operator/3, NQmin_i/1
  ILi/1 -> Compare To Constant3/1
  Compare To Constant3/1 -> Logical Operator2/2, CurrentLimit_i/1
  Logical Operator2/1 -> Logical Operator3/1
  Logical Operator/1 -> Logical Operator4/1
  Logical Operator4/1 -> Logical Operator5/1
  Logical Operator3/1 -> Logical Operator5/2
  Logical Operator5/1 -> Memory/1
  Ton_iqcot3/1 -> Compare To Constant/2

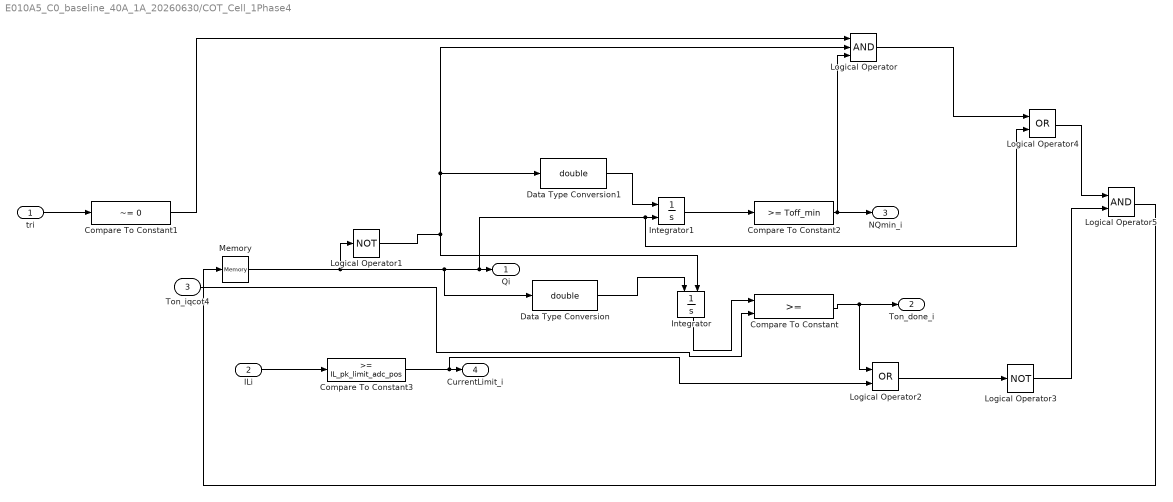
== system E010A5_C0_baseline_40A_1A_20260630/COT_Cell_1Phase4 ==
  tri : Inport
  ILi : Inport  Port=2
  Ton_iqcot4 : Inport  Port=3
  Compare To Constant : RelationalOperator  OutDataTypeStr=boolean  RndMeth=Simplest  InputSameDT=off
  Compare To Constant1 : simulink/Logic and Bit Operations/Compare To Constant  relop=~=  const=0  OutDataTypeStr=boolean
  Compare To Constant2 : simulink/Logic and Bit Operations/Compare To Constant  relop=>=  const=Toff_min  OutDataTypeStr=boolean
  Compare To Constant3 : simulink/Logic and Bit Operations/Compare To Constant  relop=>=  const=IL_pk_limit_adc_pos  OutDataTypeStr=boolean
  Data Type Conversion : DataTypeConversion  OutDataTypeStr=double  SaturateOnIntegerOverflow=off  RndMeth=Floor
  Data Type Conversion1 : DataTypeConversion  OutDataTypeStr=double  SaturateOnIntegerOverflow=off  RndMeth=Floor
  Integrator : Integrator  ExternalReset=level
  Integrator1 : Integrator  ExternalReset=level  InitialCondition=Toff_min
  Logical Operator : Logic  Inputs=3  AllPortsSameDT=off  OutDataTypeStr=boolean
  Logical Operator1 : Logic  Operator=NOT  AllPortsSameDT=off  OutDataTypeStr=boolean
  Logical Operator2 : Logic  Operator=OR  AllPortsSameDT=off  OutDataTypeStr=boolean
  Logical Operator3 : Logic  Operator=NOT  Inputs=3  AllPortsSameDT=off  OutDataTypeStr=boolean
  Logical Operator4 : Logic  Operator=OR  AllPortsSameDT=off  OutDataTypeStr=boolean
  Logical Operator5 : Logic  AllPortsSameDT=off  OutDataTypeStr=boolean
  Memory : Memory
  Qi : Outport
  Ton_done_i : Outport  Port=2
  NQmin_i : Outport  Port=3
  CurrentLimit_i : Outport  Port=4
  wires:
  Compare To Constant/1 -> Logical Operator2/1, Ton_done_i/1
  tri/1 -> Compare To Constant1/1
  Compare To Constant1/1 -> Logical Operator/1
  Memory/1 -> Logical Operator1/1, Data Type Conversion/1, Logical Operator4/2, Integrator1/2, Qi/1
  Logical Operator1/1 -> Data Type Conversion1/1, Logical Operator/2, Integrator/2
  Data Type Conversion/1 -> Integrator/1
  Integrator/1 -> Compare To Constant/1
  Data Type Conversion1/1 -> Integrator1/1
  Integrator1/1 -> Compare To Constant2/1
  Compare To Constant2/1 -> Logical Operator/3, NQmin_i/1
  ILi/1 -> Compare To Constant3/1
  Compare To Constant3/1 -> Logical Operator2/2, CurrentLimit_i/1
  Logical Operator2/1 -> Logical Operator3/1
  Logical Operator/1 -> Logical Operator4/1
  Logical Operator4/1 -> Logical Operator5/1
  Logical Operator3/1 -> Logical Operator5/2
  Logical Operator5/1 -> Memory/1
  Ton_iqcot4/1 -> Compare To Constant/2

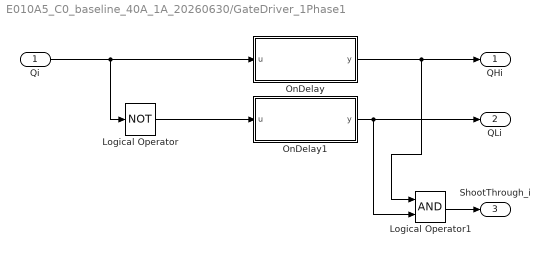
== system E010A5_C0_baseline_40A_1A_20260630/GateDriver_1Phase1 ==
  Qi : Inport
  Logical Operator : Logic  Operator=NOT  AllPortsSameDT=off  OutDataTypeStr=boolean
  Logical Operator1 : Logic  AllPortsSameDT=off  OutDataTypeStr=boolean
  OnDelay : Subsystem
  OnDelay1 : Subsystem
  QHi : Outport
  QLi : Outport  Port=2
  ShootThrough_i : Outport  Port=3
  wires:
  Qi/1 -> Logical Operator/1, OnDelay/1(u)
  OnDelay/1(y) -> Logical Operator1/1, QHi/1
  Logical Operator/1 -> OnDelay1/1(u)
  OnDelay1/1(y) -> QLi/1, Logical Operator1/2
  Logical Operator1/1 -> ShootThrough_i/1

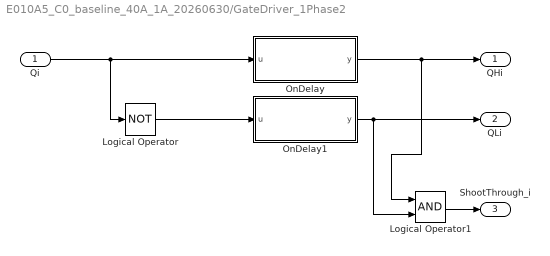
== system E010A5_C0_baseline_40A_1A_20260630/GateDriver_1Phase2 ==
  Qi : Inport
  Logical Operator : Logic  Operator=NOT  AllPortsSameDT=off  OutDataTypeStr=boolean
  Logical Operator1 : Logic  AllPortsSameDT=off  OutDataTypeStr=boolean
  OnDelay : Subsystem
  OnDelay1 : Subsystem
  QHi : Outport
  QLi : Outport  Port=2
  ShootThrough_i : Outport  Port=3
  wires:
  Qi/1 -> Logical Operator/1, OnDelay/1(u)
  OnDelay/1(y) -> Logical Operator1/1, QHi/1
  Logical Operator/1 -> OnDelay1/1(u)
  OnDelay1/1(y) -> QLi/1, Logical Operator1/2
  Logical Operator1/1 -> ShootThrough_i/1

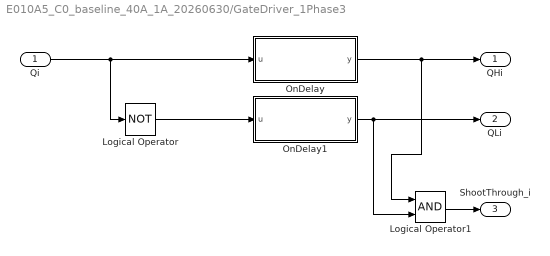
== system E010A5_C0_baseline_40A_1A_20260630/GateDriver_1Phase3 ==
  Qi : Inport
  Logical Operator : Logic  Operator=NOT  AllPortsSameDT=off  OutDataTypeStr=boolean
  Logical Operator1 : Logic  AllPortsSameDT=off  OutDataTypeStr=boolean
  OnDelay : Subsystem
  OnDelay1 : Subsystem
  QHi : Outport
  QLi : Outport  Port=2
  ShootThrough_i : Outport  Port=3
  wires:
  Qi/1 -> Logical Operator/1, OnDelay/1(u)
  OnDelay/1(y) -> Logical Operator1/1, QHi/1
  Logical Operator/1 -> OnDelay1/1(u)
  OnDelay1/1(y) -> QLi/1, Logical Operator1/2
  Logical Operator1/1 -> ShootThrough_i/1

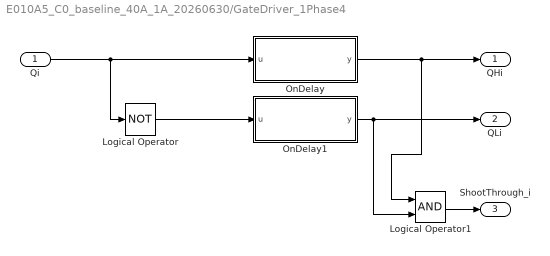
== system E010A5_C0_baseline_40A_1A_20260630/GateDriver_1Phase4 ==
  Qi : Inport
  Logical Operator : Logic  Operator=NOT  AllPortsSameDT=off  OutDataTypeStr=boolean
  Logical Operator1 : Logic  AllPortsSameDT=off  OutDataTypeStr=boolean
  OnDelay : Subsystem
  OnDelay1 : Subsystem
  QHi : Outport
  QLi : Outport  Port=2
  ShootThrough_i : Outport  Port=3
  wires:
  Qi/1 -> Logical Operator/1, OnDelay/1(u)
  OnDelay/1(y) -> Logical Operator1/1, QHi/1
  Logical Operator/1 -> OnDelay1/1(u)
  OnDelay1/1(y) -> QLi/1, Logical Operator1/2
  Logical Operator1/1 -> ShootThrough_i/1

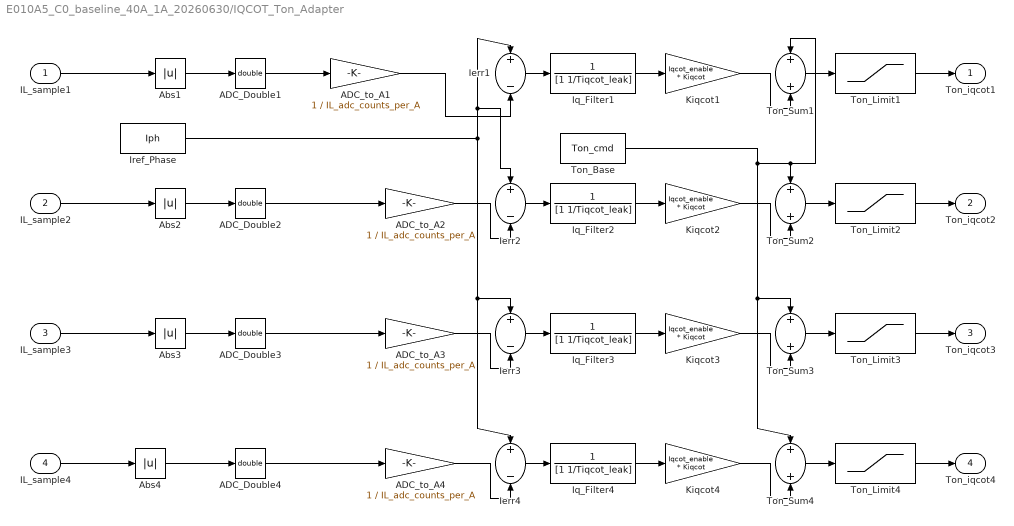
== system E010A5_C0_baseline_40A_1A_20260630/IQCOT_Ton_Adapter ==
  IL_sample1 : Inport
  IL_sample2 : Inport  Port=2
  IL_sample3 : Inport  Port=3
  IL_sample4 : Inport  Port=4
  ADC_Double{1..4} (4 alike) : DataTypeConversion  OutDataTypeStr=double  SaturateOnIntegerOverflow=off  RndMeth=Floor
  ADC_to_A{1..4} (4 alike) : Gain  Gain=1 / IL_adc_counts_per_A  OutDataTypeStr=double
  Abs{1..4} (4 alike) : Abs  SaturateOnIntegerOverflow=off
  Ierr{1..4} (4 alike) : Sum  Inputs=+-
  Iq_Filter{1..4} (4 alike) : TransferFcn  Numerator=1  Denominator=[1 1/Tiqcot_leak]
  Iref_Phase : Constant  Value=Iph
  Kiqcot{1..4} (4 alike) : Gain  Gain=Iqcot_enable * Kiqcot
  Ton_Base : Constant  Value=Ton_cmd
  Ton_Limit{1..4} (4 alike) : Saturate  UpperLimit=Ton_iq_max  LowerLimit=Ton_iq_min
  Ton_Sum{1..4} (4 alike) : Sum
  Ton_iqcot1 : Outport
  Ton_iqcot2 : Outport  Port=2
  Ton_iqcot3 : Outport  Port=3
  Ton_iqcot4 : Outport  Port=4
  wires:
  IL_sample1/1 -> Abs1/1
  Abs1/1 -> ADC_Double1/1
  ADC_to_A1/1 -> Ierr1/2
  Iref_Phase/1 -> Ierr1/1, Ierr2/1, Ierr3/1, Ierr4/1
  Ierr1/1 -> Iq_Filter1/1
  Iq_Filter1/1 -> Kiqcot1/1
  Kiqcot1/1 -> Ton_Sum1/2
  Ton_Base/1 -> Ton_Sum3/1, Ton_Sum4/1, Ton_Sum1/1, Ton_Sum2/1
  Ton_Sum1/1 -> Ton_Limit1/1
  Ton_Limit1/1 -> Ton_iqcot1/1
  IL_sample2/1 -> Abs2/1
  Abs2/1 -> ADC_Double2/1
  ADC_to_A2/1 -> Ierr2/2
  Ierr2/1 -> Iq_Filter2/1
  Iq_Filter2/1 -> Kiqcot2/1
  Kiqcot2/1 -> Ton_Sum2/2
  Ton_Sum2/1 -> Ton_Limit2/1
  Ton_Limit2/1 -> Ton_iqcot2/1
  IL_sample3/1 -> Abs3/1
  Abs3/1 -> ADC_Double3/1
  ADC_to_A3/1 -> Ierr3/2
  Ierr3/1 -> Iq_Filter3/1
  Iq_Filter3/1 -> Kiqcot3/1
  Kiqcot3/1 -> Ton_Sum3/2
  Ton_Sum3/1 -> Ton_Limit3/1
  Ton_Limit3/1 -> Ton_iqcot3/1
  IL_sample4/1 -> Abs4/1
  Abs4/1 -> ADC_Double4/1
  ADC_to_A4/1 -> Ierr4/2
  Ierr4/1 -> Iq_Filter4/1
  Iq_Filter4/1 -> Kiqcot4/1
  Kiqcot4/1 -> Ton_Sum4/2
  Ton_Sum4/1 -> Ton_Limit4/1
  Ton_Limit4/1 -> Ton_iqcot4/1
  ADC_Double1/1 -> ADC_to_A1/1
  ADC_Double2/1 -> ADC_to_A2/1
  ADC_Double3/1 -> ADC_to_A3/1
  ADC_Double4/1 -> ADC_to_A4/1

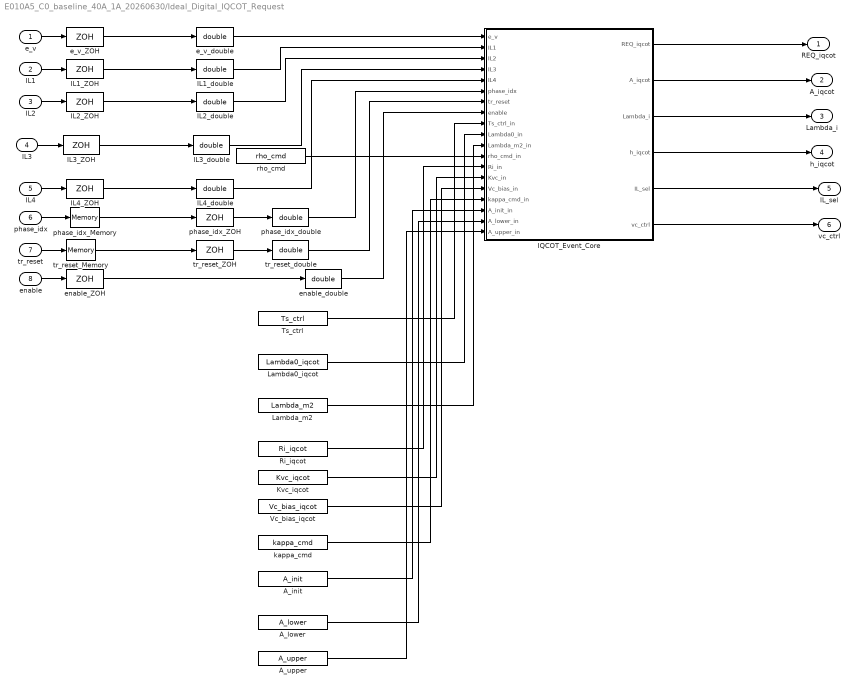
== system E010A5_C0_baseline_40A_1A_20260630/Ideal_Digital_IQCOT_Request ==
  e_v : Inport
  IL1 : Inport  Port=2
  IL2 : Inport  Port=3
  IL3 : Inport  Port=4
  IL4 : Inport  Port=5
  phase_idx : Inport  Port=6
  tr_reset : Inport  Port=7
  enable : Inport  Port=8
  A_init : Constant  Value=A_init
  A_lower : Constant  Value=A_lower
  A_upper : Constant  Value=A_upper
  IL1_ZOH : ZeroOrderHold  SampleTime=Ts_ctrl
  IL1_double : DataTypeConversion  OutDataTypeStr=double  SaturateOnIntegerOverflow=off  RndMeth=Floor
  IL2_ZOH : ZeroOrderHold  SampleTime=Ts_ctrl
  IL2_double : DataTypeConversion  OutDataTypeStr=double  SaturateOnIntegerOverflow=off  RndMeth=Floor
  IL3_ZOH : ZeroOrderHold  SampleTime=Ts_ctrl
  IL3_double : DataTypeConversion  OutDataTypeStr=double  SaturateOnIntegerOverflow=off  RndMeth=Floor
  IL4_ZOH : ZeroOrderHold  SampleTime=Ts_ctrl
  IL4_double : DataTypeConversion  OutDataTypeStr=double  SaturateOnIntegerOverflow=off  RndMeth=Floor
  IQCOT_Event_Core : MATLAB Function  TreatAsAtomicUnit=on
  Kvc_iqcot : Constant  Value=Kvc_iqcot
  Lambda0_iqcot : Constant  Value=Lambda0_iqcot
  Lambda_m2 : Constant  Value=Lambda_m2
  Ri_iqcot : Constant  Value=Ri_iqcot
  Ts_ctrl : Constant  Value=Ts_ctrl
  Vc_bias_iqcot : Constant  Value=Vc_bias_iqcot
  e_v_ZOH : ZeroOrderHold  SampleTime=Ts_ctrl
  e_v_double : DataTypeConversion  OutDataTypeStr=double  SaturateOnIntegerOverflow=off  RndMeth=Floor
  enable_ZOH : ZeroOrderHold  SampleTime=Ts_ctrl
  enable_double : DataTypeConversion  OutDataTypeStr=double  SaturateOnIntegerOverflow=off  RndMeth=Floor
  kappa_cmd : Constant  Value=kappa_cmd
  phase_idx_Memory : Memory
  phase_idx_ZOH : ZeroOrderHold  SampleTime=Ts_ctrl
  phase_idx_double : DataTypeConversion  OutDataTypeStr=double  SaturateOnIntegerOverflow=off  RndMeth=Floor
  rho_cmd : Constant  Value=rho_cmd
  tr_reset_Memory : Memory
  tr_reset_ZOH : ZeroOrderHold  SampleTime=Ts_ctrl
  tr_reset_double : DataTypeConversion  OutDataTypeStr=double  SaturateOnIntegerOverflow=off  RndMeth=Floor
  REQ_iqcot : Outport
  A_iqcot : Outport  Port=2
  Lambda_i : Outport  Port=3
  h_iqcot : Outport  Port=4
  IL_sel : Outport  Port=5
  vc_ctrl : Outport  Port=6
  wires:
  e_v/1 -> e_v_ZOH/1
  e_v_ZOH/1 -> e_v_double/1
  IL1/1 -> IL1_ZOH/1
  IL1_ZOH/1 -> IL1_double/1
  IL2/1 -> IL2_ZOH/1
  IL2_ZOH/1 -> IL2_double/1
  IL3/1 -> IL3_ZOH/1
  IL3_ZOH/1 -> IL3_double/1
  IL4/1 -> IL4_ZOH/1
  IL4_ZOH/1 -> IL4_double/1
  phase_idx/1 -> phase_idx_Memory/1
  phase_idx_Memory/1 -> phase_idx_ZOH/1
  phase_idx_ZOH/1 -> phase_idx_double/1
  tr_reset/1 -> tr_reset_Memory/1
  tr_reset_Memory/1 -> tr_reset_ZOH/1
  tr_reset_ZOH/1 -> tr_reset_double/1
  enable/1 -> enable_ZOH/1
  enable_ZOH/1 -> enable_double/1
  e_v_double/1 -> IQCOT_Event_Core/1(e_v)
  IL1_double/1 -> IQCOT_Event_Core/2(IL1)
  IL2_double/1 -> IQCOT_Event_Core/3(IL2)
  IL3_double/1 -> IQCOT_Event_Core/4(IL3)
  IL4_double/1 -> IQCOT_Event_Core/5(IL4)
  phase_idx_double/1 -> IQCOT_Event_Core/6(phase_idx)
  tr_reset_double/1 -> IQCOT_Event_Core/7(tr_reset)
  enable_double/1 -> IQCOT_Event_Core/8(enable)
  Ts_ctrl/1 -> IQCOT_Event_Core/9(Ts_ctrl_in)
  Lambda0_iqcot/1 -> IQCOT_Event_Core/10(Lambda0_in)
  Lambda_m2/1 -> IQCOT_Event_Core/11(Lambda_m2_in)
  rho_cmd/1 -> IQCOT_Event_Core/12(rho_cmd_in)
  Ri_iqcot/1 -> IQCOT_Event_Core/13(Ri_in)
  Kvc_iqcot/1 -> IQCOT_Event_Core/14(Kvc_in)
  Vc_bias_iqcot/1 -> IQCOT_Event_Core/15(Vc_bias_in)
  kappa_cmd/1 -> IQCOT_Event_Core/16(kappa_cmd_in)
  A_init/1 -> IQCOT_Event_Core/17(A_init_in)
  A_lower/1 -> IQCOT_Event_Core/18(A_lower_in)
  A_upper/1 -> IQCOT_Event_Core/19(A_upper_in)
  IQCOT_Event_Core/1(REQ_iqcot) -> REQ_iqcot/1
  IQCOT_Event_Core/2(A_iqcot) -> A_iqcot/1
  IQCOT_Event_Core/3(Lambda_i) -> Lambda_i/1
  IQCOT_Event_Core/4(h_iqcot) -> h_iqcot/1
  IQCOT_Event_Core/5(IL_sel) -> IL_sel/1
  IQCOT_Event_Core/6(vc_ctrl) -> vc_ctrl/1

== system E010A5_C0_baseline_40A_1A_20260630/OnDelay ==
  u : Inport
  Compare To Constant : simulink/Logic and Bit Operations/Compare To Constant  relop=>=  const=Tdead  OutDataTypeStr=boolean
  Data Type Conversion : DataTypeConversion  OutDataTypeStr=double  SaturateOnIntegerOverflow=off  RndMeth=Floor
  Integrator : Integrator  ExternalReset=level
  Logical Operator : Logic  Operator=NOT  AllPortsSameDT=off  OutDataTypeStr=boolean
  y : Outport
  wires:
  u/1 -> Data Type Conversion/1, Logical Operator/1
  Logical Operator/1 -> Integrator/2
  Data Type Conversion/1 -> Integrator/1
  Integrator/1 -> Compare To Constant/1
  Compare To Constant/1 -> y/1

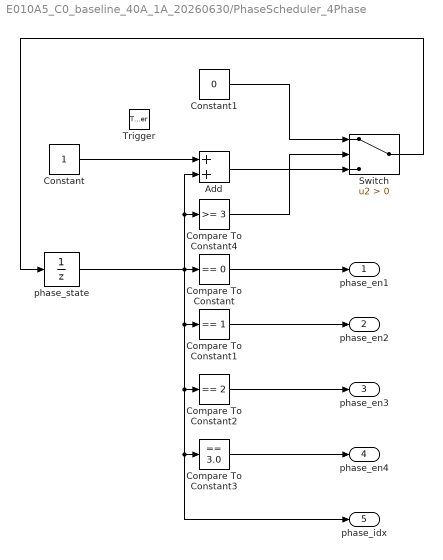
== system E010A5_C0_baseline_40A_1A_20260630/PhaseScheduler_4Phase ==
  Trigger : TriggerPort  VariantControl=(inherit)
  Add : Sum
  Compare To Constant : simulink/Logic and Bit Operations/Compare To Constant  relop===  const=0  OutDataTypeStr=boolean
  Compare To Constant1 : simulink/Logic and Bit Operations/Compare To Constant  relop===  const=1  OutDataTypeStr=boolean
  Compare To Constant2 : simulink/Logic and Bit Operations/Compare To Constant  relop===  const=2  OutDataTypeStr=boolean
  Compare To Constant3 : simulink/Logic and Bit Operations/Compare To Constant  relop===  const=3.0  OutDataTypeStr=boolean
  Compare To Constant4 : simulink/Logic and Bit Operations/Compare To Constant  relop=>=  const=3  OutDataTypeStr=boolean
  Constant : Constant
  Constant1 : Constant  Value=0
  Switch : Switch  Criteria=u2 > Threshold  SaturateOnIntegerOverflow=off  InputSameDT=off
  phase_state : UnitDelay  SampleTime=-1  HasFrameUpgradeWarning=on
  phase_en1 : Outport
  phase_en2 : Outport  Port=2
  phase_en3 : Outport  Port=3
  phase_en4 : Outport  Port=4
  phase_idx : Outport  Port=5
  wires:
  phase_state/1 -> phase_idx/1, Compare To Constant3/1, Compare To Constant2/1, Compare To Constant1/1, Compare To Constant/1, Compare To Constant4/1, Add/2
  Compare To Constant/1 -> phase_en1/1
  Compare To Constant1/1 -> phase_en2/1
  Compare To Constant2/1 -> phase_en3/1
  Compare To Constant3/1 -> phase_en4/1
  Constant/1 -> Add/1
  Add/1 -> Switch/3
  Compare To Constant4/1 -> Switch/2
  Constant1/1 -> Switch/1
  Switch/1 -> phase_state/1

== system E010A5_C0_baseline_40A_1A_20260630/GateDriver_1Phase1/OnDelay ==
  u : Inport
  Compare To Constant : simulink/Logic and Bit Operations/Compare To Constant  relop=>=  const=Tdead  OutDataTypeStr=boolean
  Data Type Conversion : DataTypeConversion  OutDataTypeStr=double  SaturateOnIntegerOverflow=off  RndMeth=Floor
  Integrator : Integrator  ExternalReset=level
  Logical Operator : Logic  Operator=NOT  AllPortsSameDT=off  OutDataTypeStr=boolean
  y : Outport
  wires:
  u/1 -> Data Type Conversion/1, Logical Operator/1
  Logical Operator/1 -> Integrator/2
  Data Type Conversion/1 -> Integrator/1
  Integrator/1 -> Compare To Constant/1
  Compare To Constant/1 -> y/1

== system E010A5_C0_baseline_40A_1A_20260630/GateDriver_1Phase1/OnDelay1 ==
  u : Inport
  Compare To Constant : simulink/Logic and Bit Operations/Compare To Constant  relop=>=  const=Tdead  OutDataTypeStr=boolean
  Data Type Conversion : DataTypeConversion  OutDataTypeStr=double  SaturateOnIntegerOverflow=off  RndMeth=Floor
  Integrator : Integrator  ExternalReset=level
  Logical Operator : Logic  Operator=NOT  AllPortsSameDT=off  OutDataTypeStr=boolean
  y : Outport
  wires:
  u/1 -> Data Type Conversion/1, Logical Operator/1
  Logical Operator/1 -> Integrator/2
  Data Type Conversion/1 -> Integrator/1
  Integrator/1 -> Compare To Constant/1
  Compare To Constant/1 -> y/1

== system E010A5_C0_baseline_40A_1A_20260630/GateDriver_1Phase2/OnDelay ==
  u : Inport
  Compare To Constant : simulink/Logic and Bit Operations/Compare To Constant  relop=>=  const=Tdead  OutDataTypeStr=boolean
  Data Type Conversion : DataTypeConversion  OutDataTypeStr=double  SaturateOnIntegerOverflow=off  RndMeth=Floor
  Integrator : Integrator  ExternalReset=level
  Logical Operator : Logic  Operator=NOT  AllPortsSameDT=off  OutDataTypeStr=boolean
  y : Outport
  wires:
  u/1 -> Data Type Conversion/1, Logical Operator/1
  Logical Operator/1 -> Integrator/2
  Data Type Conversion/1 -> Integrator/1
  Integrator/1 -> Compare To Constant/1
  Compare To Constant/1 -> y/1

== system E010A5_C0_baseline_40A_1A_20260630/GateDriver_1Phase2/OnDelay1 ==
  u : Inport
  Compare To Constant : simulink/Logic and Bit Operations/Compare To Constant  relop=>=  const=Tdead  OutDataTypeStr=boolean
  Data Type Conversion : DataTypeConversion  OutDataTypeStr=double  SaturateOnIntegerOverflow=off  RndMeth=Floor
  Integrator : Integrator  ExternalReset=level
  Logical Operator : Logic  Operator=NOT  AllPortsSameDT=off  OutDataTypeStr=boolean
  y : Outport
  wires:
  u/1 -> Data Type Conversion/1, Logical Operator/1
  Logical Operator/1 -> Integrator/2
  Data Type Conversion/1 -> Integrator/1
  Integrator/1 -> Compare To Constant/1
  Compare To Constant/1 -> y/1

== system E010A5_C0_baseline_40A_1A_20260630/GateDriver_1Phase3/OnDelay ==
  u : Inport
  Compare To Constant : simulink/Logic and Bit Operations/Compare To Constant  relop=>=  const=Tdead  OutDataTypeStr=boolean
  Data Type Conversion : DataTypeConversion  OutDataTypeStr=double  SaturateOnIntegerOverflow=off  RndMeth=Floor
  Integrator : Integrator  ExternalReset=level
  Logical Operator : Logic  Operator=NOT  AllPortsSameDT=off  OutDataTypeStr=boolean
  y : Outport
  wires:
  u/1 -> Data Type Conversion/1, Logical Operator/1
  Logical Operator/1 -> Integrator/2
  Data Type Conversion/1 -> Integrator/1
  Integrator/1 -> Compare To Constant/1
  Compare To Constant/1 -> y/1

== system E010A5_C0_baseline_40A_1A_20260630/GateDriver_1Phase3/OnDelay1 ==
  u : Inport
  Compare To Constant : simulink/Logic and Bit Operations/Compare To Constant  relop=>=  const=Tdead  OutDataTypeStr=boolean
  Data Type Conversion : DataTypeConversion  OutDataTypeStr=double  SaturateOnIntegerOverflow=off  RndMeth=Floor
  Integrator : Integrator  ExternalReset=level
  Logical Operator : Logic  Operator=NOT  AllPortsSameDT=off  OutDataTypeStr=boolean
  y : Outport
  wires:
  u/1 -> Data Type Conversion/1, Logical Operator/1
  Logical Operator/1 -> Integrator/2
  Data Type Conversion/1 -> Integrator/1
  Integrator/1 -> Compare To Constant/1
  Compare To Constant/1 -> y/1

== system E010A5_C0_baseline_40A_1A_20260630/GateDriver_1Phase4/OnDelay ==
  u : Inport
  Compare To Constant : simulink/Logic and Bit Operations/Compare To Constant  relop=>=  const=Tdead  OutDataTypeStr=boolean
  Data Type Conversion : DataTypeConversion  OutDataTypeStr=double  SaturateOnIntegerOverflow=off  RndMeth=Floor
  Integrator : Integrator  ExternalReset=level
  Logical Operator : Logic  Operator=NOT  AllPortsSameDT=off  OutDataTypeStr=boolean
  y : Outport
  wires:
  u/1 -> Data Type Conversion/1, Logical Operator/1
  Logical Operator/1 -> Integrator/2
  Data Type Conversion/1 -> Integrator/1
  Integrator/1 -> Compare To Constant/1
  Compare To Constant/1 -> y/1

== system E010A5_C0_baseline_40A_1A_20260630/GateDriver_1Phase4/OnDelay1 ==
  u : Inport
  Compare To Constant : simulink/Logic and Bit Operations/Compare To Constant  relop=>=  const=Tdead  OutDataTypeStr=boolean
  Data Type Conversion : DataTypeConversion  OutDataTypeStr=double  SaturateOnIntegerOverflow=off  RndMeth=Floor
  Integrator : Integrator  ExternalReset=level
  Logical Operator : Logic  Operator=NOT  AllPortsSameDT=off  OutDataTypeStr=boolean
  y : Outport
  wires:
  u/1 -> Data Type Conversion/1, Logical Operator/1
  Logical Operator/1 -> Integrator/2
  Data Type Conversion/1 -> Integrator/1
  Integrator/1 -> Compare To Constant/1
  Compare To Constant/1 -> y/1

== matlab function E010A5_C0_baseline_40A_1A_20260630/E010A5_SevereDropDetector ==
  data: iload input double size=1; detected output double size=1; t input double size=1; threshold input double size=1
function detected = severe_drop_detector(iload,t,threshold)
%#codegen
persistent initial_load latched
if isempty(initial_load)
    initial_load = iload;
end
if isempty(latched)
    latched = false;
end
if t < 1.0e-9
    initial_load = iload;
    latched = false;
end
if (initial_load - iload) >= threshold
    latched = true;
end
detected = double(latched);

== matlab function E010A5_C0_baseline_40A_1A_20260630/E010A5_TonActual1 ==
  data: qh input boolean size=1; Ton_actual output double size=1; t input double size=1
function Ton_actual = ton_actual_estimator(qh, t)
%#codegen
persistent q_prev t_rise last_width
if isempty(q_prev)
    q_prev = 0.0;
end
if isempty(t_rise)
    t_rise = 0.0;
end
if isempty(last_width)
    last_width = 0.0;
end
is_high = double(qh > 0.5);
if is_high > 0.5 && q_prev <= 0.5
    t_rise = t;
elseif is_high <= 0.5 && q_prev > 0.5
    last_width = max(0.0, t - t_rise);
end
Ton_actual = last_width;
q_prev = is_high;

== matlab function E010A5_C0_baseline_40A_1A_20260630/E010A5_TonActual2 ==
  data: qh input boolean size=1; Ton_actual output double size=1; t input double size=1
function Ton_actual = ton_actual_estimator(qh, t)
%#codegen
persistent q_prev t_rise last_width
if isempty(q_prev)
    q_prev = 0.0;
end
if isempty(t_rise)
    t_rise = 0.0;
end
if isempty(last_width)
    last_width = 0.0;
end
is_high = double(qh > 0.5);
if is_high > 0.5 && q_prev <= 0.5
    t_rise = t;
elseif is_high <= 0.5 && q_prev > 0.5
    last_width = max(0.0, t - t_rise);
end
Ton_actual = last_width;
q_prev = is_high;
